simulink model "PartC"  (R2019b)
settings: Solver=VariableStepAuto  StartTime=0.0  StopTime=10.0  RelTol=1e-3
settings Model: Creator=visha  LastModifiedBy=visha
settings OptimizationCC: DefaultParameterBehavior=Inlined

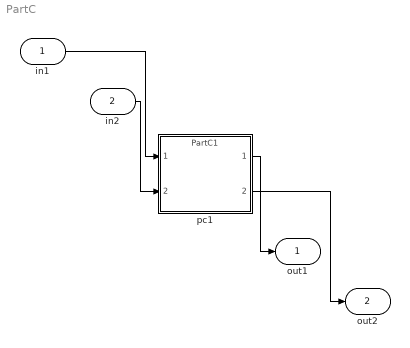
== system PartC ==
  in1 : Inport  OutDataTypeStr=double
  in2 : Inport  Port=2  OutDataTypeStr=int32
  pc1 : ModelReference  ModelNameDialog=PartC1  SimulationMode=Normal  ModelReferenceVersion=1.1
  out1 : Outport  OutDataTypeStr=double
  out2 : Outport  Port=2  OutDataTypeStr=boolean
  wires:
  in1/1 -> pc1/1
  in2/1 -> pc1/2
  pc1/1 -> out1/1
  pc1/2 -> out2/1
